simulink model "cdip_pcont_least_square_sim"  (R2013a)
settings: Solver=ode4  StartTime=0.0  StopTime=8  FixedStep=0.001  RelTol=1e-3
values from neighbouring files (symbols this model uses):
  ac = 2*zeta*omega_n    [p1c321_cdip_id_cart.m]    (also in p1c322_cdip_id_least_square.m = p1(1))
  bc = omega_n^2/kP    [p1c321_cdip_id_cart.m]    (also in p1c322_cdip_id_least_square.m = p1(2))
  dtheta_0 = 0    [p1c322_cdip_id_least_square.m]    (also in p1c34_cdip_plot_pcont.m)
  dz_0 = 0    [p1c322_cdip_id_least_square.m]    (also in p1c34_cdip_plot_pcont.m)
  g = 9.81e+000    (= 9.81)    [p1c321_cdip_id_pend.m]    (also in p1c322_cdip_id_least_square.m; p1c322_cdip_plot_MN.m; p1c332_adip_id_least_square.m; p1c332_adip_id_pend.m)
  Jp = mp*g*lp/omega_n^2 - mp*lp^2    [p1c321_cdip_id_pend.m]    (also in p1c322_cdip_id_least_square.m = p2(1))
  kP = 10    [p1c321_cdip_id_cart.m]    (also in p1c322_cdip_id_least_square.m; p1c322_cdip_plot_MN.m; p1c332_adip_id_arm.m = 3; p1c332_adip_id_least_square.m = 3)
  lp = 2.30e-001    (= 0.23)    [p1c321_cdip_id_pend.m]    (also in p1c322_cdip_id_least_square.m; p1c322_cdip_plot_MN.m)
  mp = 1.07e-001    (= 0.107)    [p1c321_cdip_id_pend.m]    (also in p1c322_cdip_id_least_square.m; p1c322_cdip_plot_MN.m)
  mup = 2*zeta*omega_n*(Jp + mp*lp^2)    [p1c321_cdip_id_pend.m]    (also in p1c322_cdip_id_least_square.m = p2(2))
  theta_0 = pi    (= 3.14159265359)    [p1c322_cdip_id_least_square.m]    (also in p1c34_cdip_plot_pcont.m)
  z_0 = 0    [p1c322_cdip_id_least_square.m]    (also in p1c34_cdip_plot_pcont.m)
settings Model: Creator=kawata  LastModifiedBy=kawata

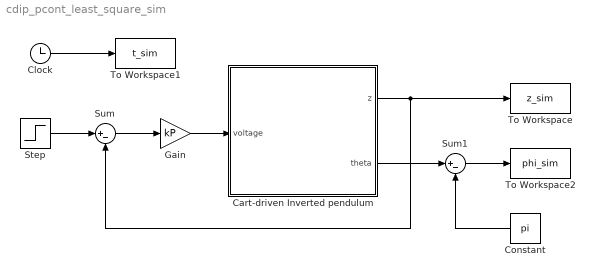
== system cdip_pcont_least_square_sim ==
  Cart-driven Inverted pendulum : Subsystem
      mask Display: image(imread('cdip.jpg'),'center')
  Clock : Clock
  Constant : Constant  Value=pi
  Gain : Gain  Gain=kP  SaturateOnIntegerOverflow=on  OutDataTypeStr=Inherit: Same as input  ParamDataTypeStr=Inherit: Same as input
  Step : Step  Time=0  After=0.2  SampleTime=0
  Sum : Sum  Inputs=|+-  SaturateOnIntegerOverflow=on  InputSameDT=on  OutDataTypeStr=Inherit: Same as first input
  Sum1 : Sum  Inputs=|+-  SaturateOnIntegerOverflow=on  InputSameDT=on  OutDataTypeStr=Inherit: Same as first input
  To Workspace : ToWorkspace  VariableName=z_sim  SampleTime=-1
  To Workspace1 : ToWorkspace  VariableName=t_sim  SampleTime=-1
  To Workspace2 : ToWorkspace  VariableName=phi_sim  SampleTime=-1
  wires:
  Cart-driven Inverted pendulum/1(z) -> To Workspace/1, Sum/2
  Step/1 -> Sum/1
  Sum/1 -> Gain/1
  Gain/1 -> Cart-driven Inverted pendulum/1(voltage)
  Clock/1 -> To Workspace1/1
  Cart-driven Inverted pendulum/2(theta) -> Sum1/1
  Sum1/1 -> To Workspace2/1
  Constant/1 -> Sum1/2

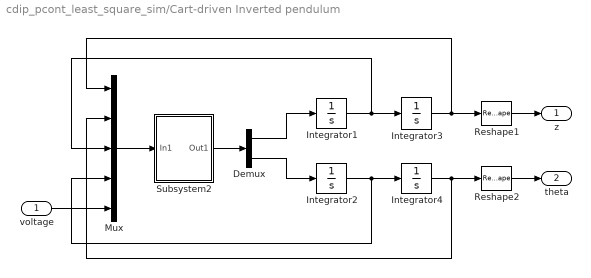
== system cdip_pcont_least_square_sim/Cart-driven Inverted pendulum ==
  voltage : Inport
  Demux : Demux  Outputs=2
  Integrator1 : Integrator  InitialCondition=dz_0
  Integrator2 : Integrator  InitialCondition=dtheta_0
  Integrator3 : Integrator  InitialCondition=z_0
  Integrator4 : Integrator  InitialCondition=theta_0
  Mux : Mux  Inputs=5
  Reshape1 : Reshape
  Reshape2 : Reshape
  Subsystem2 : Subsystem
  z : Outport
  theta : Outport  Port=2
  wires:
  Subsystem2/1(Out1) -> Demux/1
  Mux/1 -> Subsystem2/1(In1)
  Demux/1 -> Integrator1/1
  Demux/2 -> Integrator2/1
  Integrator1/1 -> Mux/3, Integrator3/1
  Integrator2/1 -> Mux/4, Integrator4/1
  Integrator3/1 -> Reshape1/1, Mux/1
  Integrator4/1 -> Reshape2/1, Mux/2
  voltage/1 -> Mux/5
  Reshape1/1 -> z/1
  Reshape2/1 -> theta/1

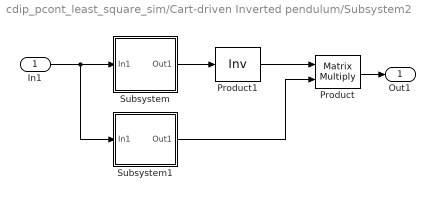
== system cdip_pcont_least_square_sim/Cart-driven Inverted pendulum/Subsystem2 ==
  In1 : Inport
  Product : Product  Multiplication=Matrix(*)  SaturateOnIntegerOverflow=on  InputSameDT=on  OutDataTypeStr=Inherit: Same as first input
  Product1 : Product  Inputs=/  Multiplication=Matrix(*)  SaturateOnIntegerOverflow=on  InputSameDT=on  OutDataTypeStr=Inherit: Same as first input
  Subsystem : Subsystem
  Subsystem1 : Subsystem
  Out1 : Outport
  wires:
  Product/1 -> Out1/1
  In1/1 -> Subsystem1/1(In1), Subsystem/1(In1)
  Subsystem1/1(Out1) -> Product/2
  Product1/1 -> Product/1
  Subsystem/1(Out1) -> Product1/1

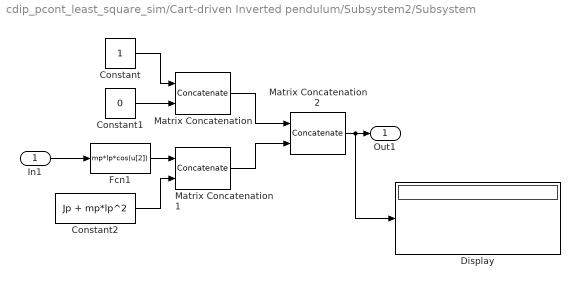
== system cdip_pcont_least_square_sim/Cart-driven Inverted pendulum/Subsystem2/Subsystem ==
  In1 : Inport
  Constant : Constant
  Constant1 : Constant  Value=0
  Constant2 : Constant  Value=Jp + mp*lp^2
  Display : Display
  Fcn1 : Fcn  Expr=mp*lp*cos(u[2])
  Matrix Concatenation : Concatenate  Mode=Multidimensional array  ConcatenateDimension=2
  Matrix Concatenation1 : Concatenate  Mode=Multidimensional array  ConcatenateDimension=2
  Matrix Concatenation2 : Concatenate  Mode=Multidimensional array
  Out1 : Outport
  wires:
  Constant1/1 -> Matrix Concatenation/2
  Constant/1 -> Matrix Concatenation/1
  Matrix Concatenation2/1 -> Out1/1, Display/1
  Matrix Concatenation1/1 -> Matrix Concatenation2/2
  Matrix Concatenation/1 -> Matrix Concatenation2/1
  In1/1 -> Fcn1/1
  Fcn1/1 -> Matrix Concatenation1/1
  Constant2/1 -> Matrix Concatenation1/2

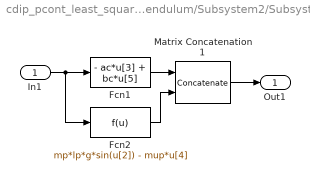
== system cdip_pcont_least_square_sim/Cart-driven Inverted pendulum/Subsystem2/Subsystem1 ==
  In1 : Inport
  Fcn1 : Fcn  Expr=- ac*u[3] + bc*u[5]
  Fcn2 : Fcn  Expr=mp*lp*g*sin(u[2]) - mup*u[4]
  Matrix Concatenation1 : Concatenate  Mode=Multidimensional array
  Out1 : Outport
  wires:
  Matrix Concatenation1/1 -> Out1/1
  In1/1 -> Fcn1/1, Fcn2/1
  Fcn1/1 -> Matrix Concatenation1/1
  Fcn2/1 -> Matrix Concatenation1/2
